simulink model "Directional_Relay"  (R2017a)
settings: Solver=VariableStepAuto  StartTime=0.0  StopTime=2  RelTol=1e-3
libraries: sdolib x6, simulink_extras x3
settings Model: Creator=ikon  LastModifiedBy=ikon

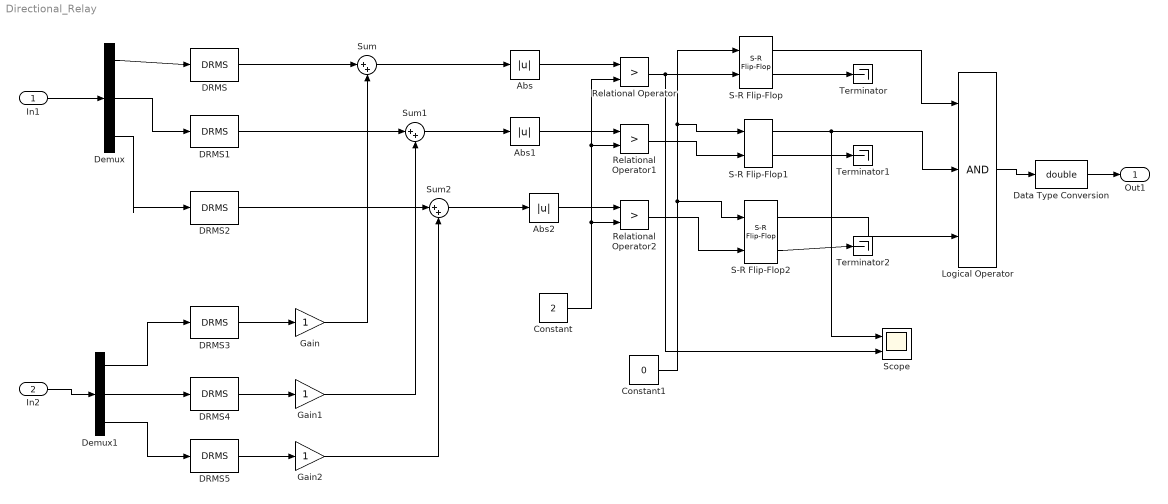
== system Directional_Relay ==
  In1 : Inport
  In2 : Inport  Port=2
  Abs : Abs
  Abs1 : Abs
  Abs2 : Abs
  Constant : Constant  Value=2
  Constant1 : Constant  Value=0
  DRMS{,1..5} (6 alike) : sdolib/RMS Blocks/DRMS  Ts=1
      settings: SourceProductName=Simulink Design Optimization  SourceProductBaseCode=SO
  Data Type Conversion : DataTypeConversion  OutDataTypeStr=double
  Demux : Demux  Outputs=3
  Demux1 : Demux  Outputs=3
  Gain : Gain
  Gain1 : Gain
  Gain2 : Gain
  Logical Operator : Logic  Inputs=3  AllPortsSameDT=off  OutDataTypeStr=boolean
  Relational Operator : RelationalOperator  Operator=>  OutDataTypeStr=boolean  RndMeth=Simplest
  Relational Operator1 : RelationalOperator  Operator=>  OutDataTypeStr=boolean  RndMeth=Simplest
  Relational Operator2 : RelationalOperator  Operator=>  OutDataTypeStr=boolean  RndMeth=Simplest
  S-R Flip-Flop : simulink_extras/Flip Flops/S-R Flip-Flop  initial_condition=0
  S-R Flip-Flop1 : simulink_extras/Flip Flops/S-R Flip-Flop  initial_condition=0
  S-R Flip-Flop2 : simulink_extras/Flip Flops/S-R Flip-Flop  initial_condition=0
  Scope : Scope  NumInputPorts=2
  Sum : Sum  Inputs=|++
  Sum1 : Sum  Inputs=|++
  Sum2 : Sum  Inputs=|++
  Terminator : Terminator
  Terminator1 : Terminator
  Terminator2 : Terminator
  Out1 : Outport
  wires:
  Demux/1 -> DRMS/1
  Demux/2 -> DRMS1/1
  Demux/3 -> DRMS2/1
  Demux1/1 -> DRMS3/1
  Demux1/2 -> DRMS4/1
  Demux1/3 -> DRMS5/1
  DRMS3/1 -> Gain/1
  DRMS4/1 -> Gain1/1
  DRMS5/1 -> Gain2/1
  DRMS2/1 -> Sum2/1
  DRMS1/1 -> Sum1/1
  DRMS/1 -> Sum/1
  Gain/1 -> Sum/2
  Gain1/1 -> Sum1/2
  Gain2/1 -> Sum2/2
  Sum/1 -> Abs/1
  Sum1/1 -> Abs1/1
  Sum2/1 -> Abs2/1
  Abs2/1 -> Relational Operator2/1
  Abs1/1 -> Relational Operator1/1
  Abs/1 -> Relational Operator/1
  Constant/1 -> Relational Operator2/2, Relational Operator1/2, Relational Operator/2
  Relational Operator/1 -> Scope/2, S-R Flip-Flop/2
  Relational Operator1/1 -> S-R Flip-Flop1/2
  Relational Operator2/1 -> S-R Flip-Flop2/2
  Constant1/1 -> S-R Flip-Flop2/1, S-R Flip-Flop1/1, S-R Flip-Flop/1
  S-R Flip-Flop/2 -> Terminator/1
  S-R Flip-Flop1/2 -> Terminator1/1
  S-R Flip-Flop2/2 -> Terminator2/1
  S-R Flip-Flop/1 -> Logical Operator/1
  S-R Flip-Flop1/1 -> Scope/1, Logical Operator/2
  S-R Flip-Flop2/1 -> Logical Operator/3
  Logical Operator/1 -> Data Type Conversion/1
  Data Type Conversion/1 -> Out1/1
  In1/1 -> Demux/1
  In2/1 -> Demux1/1
